simulink model "MPC_UPS"  (R2019a)
settings: Solver=VariableStepAuto  StartTime=0.0  StopTime=0.1  RelTol=1e-3
undefined symbols (not defined in the file or in its folder): C, L, R, Vdc
libraries: powerlib x12
settings Model: Creator=Vu Hung Dung  LastModifiedBy=Vu Hung Dung
settings DataIOCC: ReturnWorkspaceOutputs=off

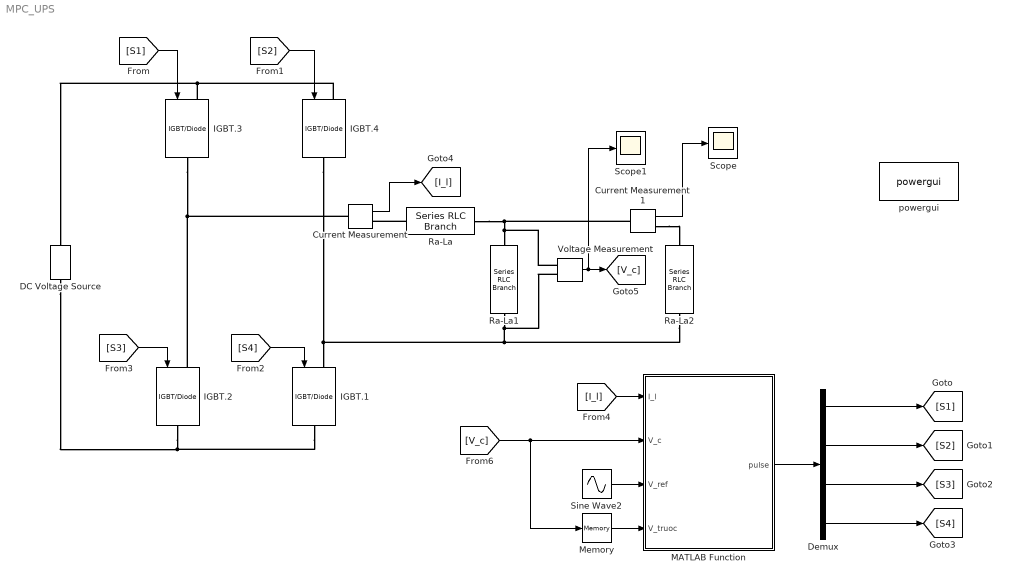
== system MPC_UPS ==
  Current Measurement : powerlib/Measurements/Current Measurement  PhasorSimulation=off  OutputType=Complex  PSBequivalent=0
      settings: SourceProductName=Simscape Electrical
  Current Measurement1 : powerlib/Measurements/Current Measurement  PhasorSimulation=off  OutputType=Complex  PSBequivalent=0
      settings: SourceProductName=Simscape Electrical
  DC Voltage Source : powerlib/Electrical Sources/DC Voltage Source  Amplitude=Vdc  Measurements=Voltage
      settings: SourceProductName=Simscape Electrical
  Demux : Demux
  IGBT.{1..4} (4 alike) : powerlib/Power Electronics/IGBT//Diode  Ron=1e-3  Rs=1e5  Cs=inf  Measurements=off
      settings: SourceProductName=Simscape Electrical
  MATLAB Function : MATLAB Function  TreatAsAtomicUnit=on
  Memory : Memory
  Ra-La : powerlib/Elements/Series RLC Branch  LConnTagsString=__new0  RConnTagsString=__new0  BranchType=L  Resistance=R  Inductance=L  SetiL0=off  InitialCurrent=0  Capacitance=1.0  Setx0=off  InitialVoltage=0  Measurements=None
      settings: SourceProductName=Simscape Electrical
  Ra-La1 : powerlib/Elements/Series RLC Branch  LConnTagsString=__new0  RConnTagsString=__new0  BranchType=C  Resistance=R  Inductance=L  SetiL0=off  InitialCurrent=0  Capacitance=C  Setx0=off  InitialVoltage=0  Measurements=None
      settings: SourceProductName=Simscape Electrical
  Ra-La2 : powerlib/Elements/Series RLC Branch  LConnTagsString=__new0  RConnTagsString=__new0  BranchType=R  Resistance=R  Inductance=L  SetiL0=off  InitialCurrent=0  Capacitance=C  Setx0=off  InitialVoltage=0  Measurements=None
      settings: SourceProductName=Simscape Electrical
  Scope : Scope
  Scope1 : Scope
  Sine Wave2 : Sin  Amplitude=100  Frequency=100*pi  SampleTime=1e-6
  Voltage Measurement : powerlib/Measurements/Voltage Measurement  PhasorSimulation=off  OutputType=Complex  PSBequivalent=0
      settings: SourceProductName=Simscape Electrical
  powergui : powerlib/powergui  Priority=1  SimulationMode=Discrete  SampleTime=1e-6  frequency=60  Iterations=50  frequencyindice=0  Pbase=100e6  ErrMax=1e-4  UnitsV=kV  UnitsW=MW  buscounter=0  FunctionMessages=off  echomessages=off  EnableUseOfTLC=off  CurrentSourceSwitches=off  DisableSnubberDevices=off  DisableRonSwitches=off  DisableVfSwitches=off  DisplayEquations=off  AutomaticDiscreteSolvers=off  SolverType=Tustin/Backward Euler (TBE)  Interpol=off  ExternalGateDelay=off  methode=off  Ts=100  x0status=blocks  SPID=on  SwTol=0  HookPort=off  NonlinearTolerance=0  nMaxIteration=15  ContinueOnMaxIteration=off  RestoreLinks=warning  ResistiveCurrentMeasurement=off  Frange=[0:2:500]  Ylog=off  Xlog=on  ShowGrid=off  save=off  variable=ZData  structure=Current  ZoomFFT=off  StartTime=0.0  cycles=1  DisplayStyle=1  fundamental=50  FreqAxis=on  MaxFrequency=1000  frequencyindicesteady=1  RmsSteady=1  display=off
      settings: SourceProductName=Simscape Electrical
  wires:
  [I_l] -> MATLAB Function/1(I_l)
  Demux/4 -> [S4]
  Demux/1 -> [S1]
  [S3] -> IGBT.2/1
  Demux/2 -> [S2]
  Current Measurement/1 -> [I_l]
  Demux/3 -> [S3]
  MATLAB Function/1(pulse) -> Demux/1
  [S4] -> IGBT.1/1
  [S2] -> IGBT.4/1
  [S1] -> IGBT.3/1
  Voltage Measurement/1 -> Scope1/1, [V_c]
  [V_c] -> MATLAB Function/2(V_c), Memory/1
  Sine Wave2/1 -> MATLAB Function/3(V_ref)
  Memory/1 -> MATLAB Function/4(V_truoc)
  Current Measurement1/1 -> Scope/1
  connections:
  IGBT.2/RConn1 -- DC Voltage Source/LConn1 -- IGBT.1/RConn1
  IGBT.4/RConn1 -- Voltage Measurement/LConn2 -- Ra-La1/RConn1 -- Ra-La2/RConn1 -- IGBT.1/LConn1
  IGBT.3/LConn1 -- DC Voltage Source/RConn1 -- IGBT.4/LConn1
  IGBT.3/RConn1 -- IGBT.2/LConn1 -- Current Measurement/LConn1
  Ra-La/LConn1 -- Current Measurement/RConn1
  Ra-La/RConn1 -- Current Measurement1/LConn1 -- Voltage Measurement/LConn1 -- Ra-La1/LConn1
  Current Measurement1/RConn1 -- Ra-La2/LConn1

== matlab function MPC_UPS/MATLAB Function ==
  data: I_l input; pulse output; V_c input; V_ref input; V_truoc input
function pulse  = MPC(I_l, V_c, V_ref, V_truoc)

L = 1e-1;
R = 10;
C = 1e-3;
Vdc = 200;
Ts = 1e-6;
S1_opt = 0;
S2_opt = 0;
g_opt = inf;

for S1 = 0:1
    for S2 = 0:1
        U1 = S1*Vdc;
        U2 = S2*Vdc;
        U = U1-U2;
        I_0 = I_l- (C/Ts)*(V_c-V_truoc);
        I_l1 = I_l+(Ts/L)*(U-V_c);
        V_dubao = V_c+(Ts/C)*(I_l1-I_0);
        g = abs(V_dubao-V_ref);
    if (g < g_opt) 
        S1_opt = S1;
        S2_opt = S2;
        g_opt = g;
    end
    end  
end
S1 = S1_opt;
S2 = S2_opt;
pulse = [S1; S2; not(S1); not(S2)];
